simulink model "MLIB_Norm_BAM_F32"  (Simulink 7.3)
settings: Solver=ode45  StartTime=0.0  StopTime=10.0  RelTol=1e-3
settings Model: Creator=B17364  LastModifiedBy=B17364

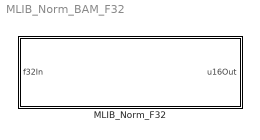
== system MLIB_Norm_BAM_F32 ==
  MLIB_Norm_F32 : Subsystem  mask(MLIB_Norm_F32){}
      mask help: Bit accurate model of the normalization function. The function counts the number of left shift needed for normalization of the input fractional value.
      mask init:
      | pos = get_param(gcb, 'Position');width = pos(3) - pos(1); height = pos(4) - pos(2);tX=width/2;tY=height*0.9;
      mask Display: color('black');port_label('input',1,'f32In');port_label('output',1,'u16Out');color('black');disp('MLIB_Norm_F32');color('blue');text(tX,tY, 'BAM', 'horizontalAlignment', 'center');

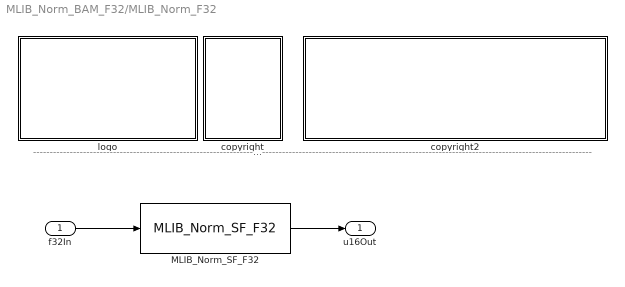
== system MLIB_Norm_BAM_F32/MLIB_Norm_F32 ==
  note: ---------------------------------------------------------------------------------------------------------------------------------------------------------------------------------------------------
  f32In : Inport  OutDataType=fixdt(1, 16)  OutScaling=2^0
  MLIB_Norm_SF_F32 : S-Function  FunctionName=MLIB_Norm_SF_F32  EnableBusSupport=off
  copyright : Subsystem
      mask Display: text(10,90,'FILE:');text(10,75,'DESRIPTION:')text(10,60,'COPYRIGHT:')text(10,45,'VERSION:')text(10,30,'DATE:')
  copyright2 : Subsystem
      mask Display: text(10,90,'MLIB_Norm_BAM_F32.mdl');text(10,75,'Normalization of the input value.');text(10,60,'Freescale')text(10,45,'0.1');text(10,30,'15-Sep-2011');
  logo : Subsystem
      mask Display: image(imread('logo.jpg'))
  u16Out : Outport  OutDataType=fixdt(1, 16)  OutScaling=2^0
  wires:
  f32In/1 -> MLIB_Norm_SF_F32/1
  MLIB_Norm_SF_F32/1 -> u16Out/1

== system MLIB_Norm_BAM_F32/MLIB_Norm_F32/copyright ==

== system MLIB_Norm_BAM_F32/MLIB_Norm_F32/copyright2 ==

== system MLIB_Norm_BAM_F32/MLIB_Norm_F32/logo ==
